simulink model "State_observer_v22b"  (R2022b)
settings: Solver=VariableStepAuto  StartTime=0.0  StopTime=30  RelTol=1e-3
undefined symbols (not defined in the file): A, alfa, B, beta, C, D, g0, Ip, Ir, Ir_tot, K, L_kf, L_pp, La, Ld, Lp, Lr, mp, mr, phi_dot_init, phi_init, Ra, rot_pend, theta_dot_init, theta_init
libraries: simulink_extras x5
settings Model: Creator=Mark  LastModifiedBy=Mark
settings OptimizationCC: ReuseModelBlockBuffer=on

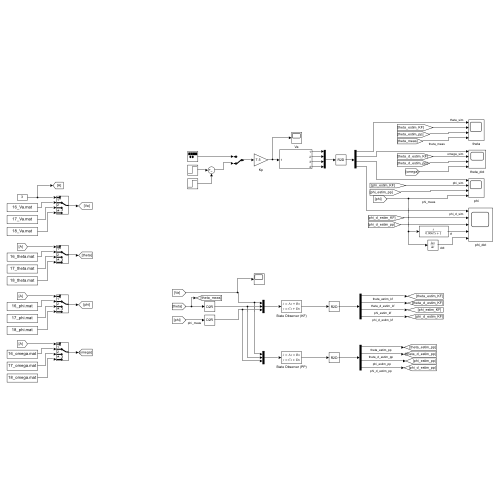
[thumbnail: Simulink's stored preview of the top-level diagram]
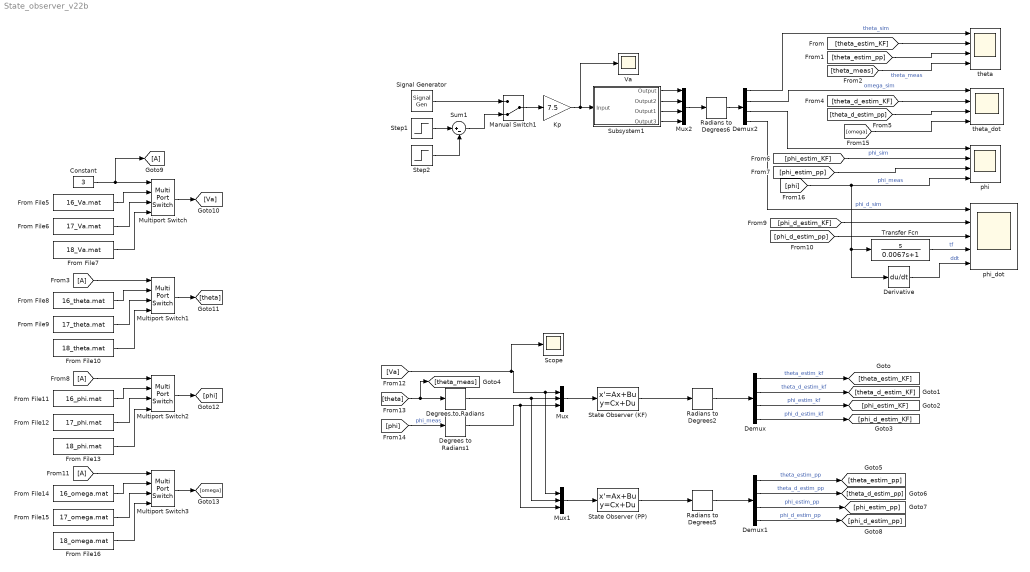
== system State_observer_v22b ==
  Constant : Constant  Value=3
  Degrees to Radians : simulink_extras/Transformations/Degrees to Radians
  Degrees to Radians1 : simulink_extras/Transformations/Degrees to Radians
  Demux : Demux
  Demux1 : Demux
  Demux2 : Demux
  Derivative : Derivative  CoefficientInTFapproximation=0.0067
  From File10 : FromFile  FileName=18_theta.mat  SampleTime=0
  From File11 : FromFile  FileName=16_phi.mat  SampleTime=0
  From File12 : FromFile  FileName=17_phi.mat  SampleTime=0
  From File13 : FromFile  FileName=18_phi.mat  SampleTime=0
  From File14 : FromFile  FileName=16_omega.mat  SampleTime=0
  From File15 : FromFile  FileName=17_omega.mat  SampleTime=0
  From File16 : FromFile  FileName=18_omega.mat  SampleTime=0
  From File5 : FromFile  FileName=16_Va.mat  SampleTime=0
  From File6 : FromFile  FileName=17_Va.mat  SampleTime=0
  From File7 : FromFile  FileName=18_Va.mat  SampleTime=0
  From File8 : FromFile  FileName=16_theta.mat  SampleTime=0
  From File9 : FromFile  FileName=17_theta.mat  SampleTime=0
  From11 : From
  From3 : From
  From8 : From
  Goto9 : Goto
  Kp : Gain  Gain=7.5
  Manual Switch1 : ManualSwitch  CurrentSetting=0
  Multiport Switch{,1..3} (4 alike) : MultiPortSwitch  SaturateOnIntegerOverflow=off  InputSameDT=off
  Mux : Mux  Inputs=3
  Mux1 : Mux  Inputs=3
  Mux2 : Mux
  Radians to Degrees2 : simulink_extras/Transformations/Radians to Degrees
  Radians to Degrees5 : simulink_extras/Transformations/Radians to Degrees
  Radians to Degrees6 : simulink_extras/Transformations/Radians to Degrees
  Scope : Scope
  Signal Generator : SignalGenerator  WaveForm=square  Frequency=0.05
  State Observer (KF) : StateSpace  A=A-L_kf*C  B=[B-L_kf*D L_kf]  C=eye(4)  D=zeros(4,3)  InitialCondition=0  ParameterTunability=Unconstrained
  State Observer (PP) : StateSpace  A=A-L_pp*C  B=[B-L_pp*D L_pp]  C=eye(4)  D=zeros(4,3)  InitialCondition=0
  Step1 : Step  SampleTime=0
  Step2 : Step  Time=1.05  SampleTime=0
  Subsystem1 : Subsystem
  Sum1 : Sum  Inputs=|+-
  Transfer Fcn : TransferFcn  Numerator=[1 0]  Denominator=[0.0067 1]
  Va : Scope
  phi : Scope  NumInputPorts=4
  phi_dot : Scope  NumInputPorts=5
  theta : Scope  NumInputPorts=4
  theta_dot : Scope  NumInputPorts=4
  wires:
  Signal Generator/1 -> Manual Switch1/1
  Manual Switch1/1 -> Kp/1
  Kp/1 -> Va/1, Subsystem1/1(Input)
  Demux/1 -> [theta_estim_KF]  "theta_estim_kf"
  Demux/2 -> [theta_d_estim_KF]  "theta_d_estim_kf"
  Demux/3 -> [phi_estim_KF]  "phi_estim_kf"
  Demux/4 -> [phi_d_estim_KF]  "phi_d_estim_kf"
  Radians to Degrees2/1 -> Demux/1
  State Observer (KF)/1 -> Radians to Degrees2/1
  Step1/1 -> Sum1/1
  Sum1/1 -> Manual Switch1/2
  Step2/1 -> Sum1/2
  Mux/1 -> State Observer (KF)/1
  [theta] -> Degrees to Radians/1, [theta_meas]
  [phi] -> Degrees to Radians1/1  "phi_meas"
  [Va] -> Scope/1, Mux1/1, Mux/1
  Degrees to Radians/1 -> Mux1/2, Mux/2
  Degrees to Radians1/1 -> Mux1/3, Mux/3
  Mux1/1 -> State Observer (PP)/1
  State Observer (PP)/1 -> Radians to Degrees5/1
  Radians to Degrees5/1 -> Demux1/1
  Demux1/1 -> [theta_estim_pp]  "theta_estim_pp"
  Demux1/2 -> [theta_d_estim_pp]  "theta_d_estim_pp"
  Demux1/3 -> [phi_estim_pp]  "phi_estim_pp"
  Demux1/4 -> [phi_d_estim_pp]  "phi_d_estim_pp"
  Subsystem1/1(Output) -> Mux2/1
  Subsystem1/3(Output1) -> Mux2/3
  Subsystem1/2(Output2) -> Mux2/2
  Subsystem1/4(Output3) -> Mux2/4
  Radians to Degrees6/1 -> Demux2/1
  Mux2/1 -> Radians to Degrees6/1
  Demux2/1 -> theta/1  "theta_sim"
  [theta_estim_KF] -> theta/2
  [theta_estim_pp] -> theta/3
  [theta_meas] -> theta/4  "theta_meas"
  Demux2/2 -> theta_dot/1  "omega_sim"
  [theta_d_estim_KF] -> theta_dot/2
  [theta_d_estim_pp] -> theta_dot/3
  [omega] -> theta_dot/4
  Demux2/3 -> phi/1  "phi_sim"
  [phi_estim_KF] -> phi/2
  [phi_estim_pp] -> phi/3
  [phi] -> phi/4, Transfer Fcn/1, Derivative/1  "phi_meas"
  Demux2/4 -> phi_dot/1  "phi_d_sim"
  [phi_d_estim_KF] -> phi_dot/2
  [phi_d_estim_pp] -> phi_dot/3
  Transfer Fcn/1 -> phi_dot/4  "tf"
  Derivative/1 -> phi_dot/5  "ddt"
  From File5/1 -> Multiport Switch/2
  From File6/1 -> Multiport Switch/3
  From File7/1 -> Multiport Switch/4
  Constant/1 -> Goto9/1, Multiport Switch/1
  From File8/1 -> Multiport Switch1/2
  From File10/1 -> Multiport Switch1/4
  From File9/1 -> Multiport Switch1/3
  From File11/1 -> Multiport Switch2/2
  From File13/1 -> Multiport Switch2/4
  From File12/1 -> Multiport Switch2/3
  From File14/1 -> Multiport Switch3/2
  From File16/1 -> Multiport Switch3/4
  From File15/1 -> Multiport Switch3/3
  From3/1 -> Multiport Switch1/1
  From8/1 -> Multiport Switch2/1
  From11/1 -> Multiport Switch3/1
  Multiport Switch/1 -> [Va]
  Multiport Switch1/1 -> [theta]
  Multiport Switch2/1 -> [phi]
  Multiport Switch3/1 -> [omega]

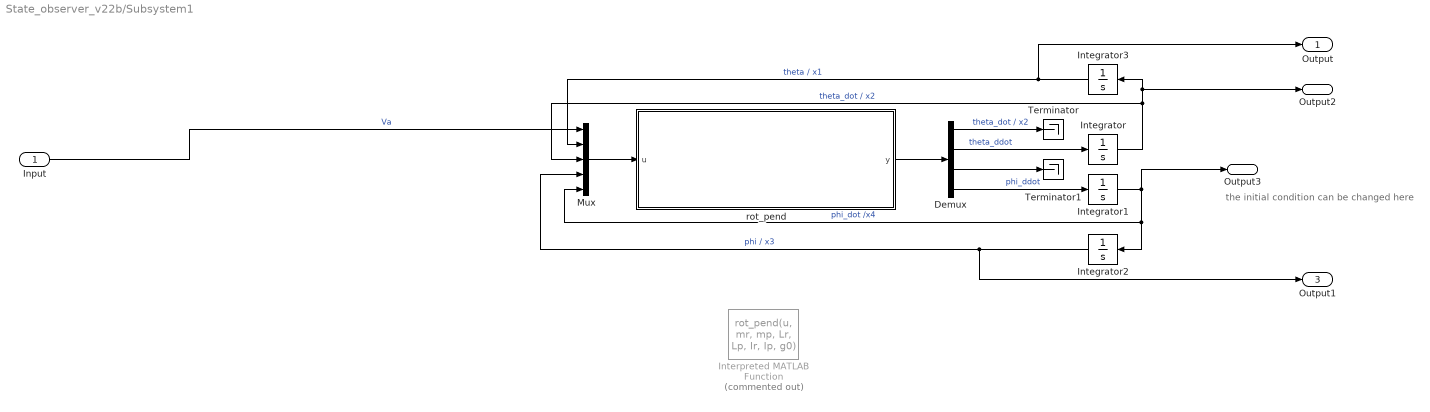
== system State_observer_v22b/Subsystem1 ==
  note: the initial condition can be changed here
  Input : Inport
  Demux : Demux
  Integrator : Integrator  InitialCondition=theta_dot_init
  Integrator1 : Integrator  InitialCondition=phi_dot_init
  Integrator2 : Integrator  InitialCondition=phi_init
  Integrator3 : Integrator  InitialCondition=theta_init
  Interpreted MATLAB Function : MATLABFcn  Commented=on  MATLABFcn=rot_pend(u, mr, mp, Lr, Lp, Ir, Ip, g0)  OutputDimensions=4  OutputSignalType=real
  Mux : Mux  Inputs=5
  Terminator : Terminator
  Terminator1 : Terminator
  rot_pend : Subsystem
  Output : Outport
  Output2 : Outport  Port=2
  Output1 : Outport  Port=3
  Output3 : Outport  Port=4
  wires:
  Integrator2/1 -> Output1/1, Mux/4  "phi / x3"
  Integrator/1 -> Integrator3/1, Output2/1, Mux/3  "theta_dot / x2"
  Mux/1 -> rot_pend/1(u)
  rot_pend/1(y) -> Demux/1
  Integrator1/1 -> Output3/1, Mux/5, Integrator2/1  "phi_dot /x4"
  Integrator3/1 -> Mux/2, Output/1  "theta / x1"
  Demux/4 -> Integrator1/1  "phi_ddot"
  Demux/2 -> Integrator/1  "theta_ddot"
  Demux/1 -> Terminator/1  "theta_dot / x2"
  Demux/3 -> Terminator1/1
  Input/1 -> Mux/1  "Va"

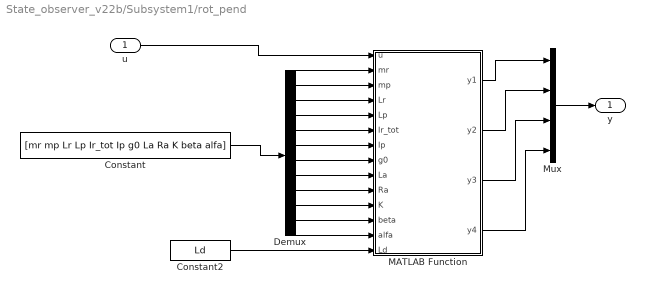
== system State_observer_v22b/Subsystem1/rot_pend ==
  u : Inport
  Constant : Constant  Value=[mr mp Lr Lp Ir_tot Ip g0 La Ra K beta alfa]  VectorParams1D=off
  Constant2 : Constant  Value=Ld
  Demux : Demux  Outputs=12
  MATLAB Function : MATLAB Function  TreatAsAtomicUnit=on
  Mux : Mux
  y : Outport
  wires:
  Demux/3 -> MATLAB Function/4(Lr)
  Demux/5 -> MATLAB Function/6(Ir_tot)
  Demux/4 -> MATLAB Function/5(Lp)
  Demux/7 -> MATLAB Function/8(g0)
  Demux/2 -> MATLAB Function/3(mp)
  Demux/6 -> MATLAB Function/7(Ip)
  Demux/1 -> MATLAB Function/2(mr)
  u/1 -> MATLAB Function/1(u)
  Constant/1 -> Demux/1
  MATLAB Function/1(y1) -> Mux/1
  MATLAB Function/2(y2) -> Mux/2
  MATLAB Function/3(y3) -> Mux/3
  MATLAB Function/4(y4) -> Mux/4
  Mux/1 -> y/1
  Demux/8 -> MATLAB Function/9(La)
  Demux/9 -> MATLAB Function/10(Ra)
  Demux/10 -> MATLAB Function/11(K)
  Demux/11 -> MATLAB Function/12(beta)
  Constant2/1 -> MATLAB Function/14(Ld)
  Demux/12 -> MATLAB Function/13(alfa)

== matlab function State_observer_v22b/Subsystem1/rot_pend/MATLAB Function ==
  data: u input; y1 output; mr input; mp input; Lr input; Lp input; Ir_tot input; Ip input; g0 input; La input; Ra input; y2 output; y3 output; y4 output; K input; beta input; alfa input; Ld input
function [y1,y2,y3,y4] = rot_pend(u, mr, mp, Lr, Lp, Ir_tot, Ip, g0,La, Ra, K, beta,alfa, Ld)
%UNTITLED Summary of this function goes here
%   Detailed explanation goes here
% u(1) = Va
x1 = u(2) ; % theta
x2 = u(3) ; % theta_dot
x3 = u(4) ; % phi
x4 = u(5) ; % phi_dot

H = [(mp*(Lr^2+((Lp/2)^2*(sin(x3))^2)))+Ir_tot            -mp*Lr*Lp*cos(x3)/2;
                     -mp*Lr*Lp*cos(x3)/2                              (mp*(Lp/2)^2)+Ip] ;

Q = [mp*(Lp/2)^2*sin(x3)*cos(x3)*x4+beta                     (mp*(Lp/2)^2*sin(x3)*cos(x3)*x2)-(mp*Lr*(Lp/2)*sin(x3)*x4);
     -mp*(Lp/2)^2*sin(x3)*cos(x3)*x2                                                   alfa                                   ] ;

g = [           0     ;
     mp*g0*(Lp/2)*sin(x3)] ;
%(K*u(1)/Ra)-(K^2*x2/Ra)
tau = [(K/Ra)*(u(1)-(K*x2)) ;
       0 ] ;

if (x1>=0.1745 | x1<=-0.1745)       % 0.08727rad = 5deg
     kt = 0.03 ;                    % 0.1745rad = 10deg
     kc = 10e-3 ;
else                               % 0.349rad = 20deg
    kt = 0 ;
    kc = 3.5e-3 ;
end
% if (x2>=2.618 | x2<=-2.618)       % 3.49rad/s = 200deg/s
%                                 % 2.618rad/s = 150deg/s
%     kc = 10e-3 ;
% else                               
% 
%     kc = 4.8e-3 ;
% end


Tr_theta = ((kt*x1)+(kc*x2))*Ld ;
q_ddot = H\[tau - Q*[x2 x4]' - g - [Tr_theta 0]' ] ;



y1 = x2 ;
y2 = q_ddot(1) ;
y3 = x4 ;
y4 = q_ddot(2) ;


%Ir+mr*(Lr/2)^2)
